simulink model "sim_5_dc_refer"  (R2022b)
settings: Solver=VariableStepAuto  StartTime=0.0  StopTime=10.0  RelTol=1e-3
model workspace: external: MAT-File dc_params.mat (data not in the file)
values from neighbouring files (symbols this model uses):
  b = 0.2    [dc_params.mat]    (also in sim_5_dc_param.m)
  J = 0.02    [dc_params.mat]    (also in sim_5_dc_param.m)
  K_e = 0.1    [dc_params.mat]    (also in sim_5_dc_param.m)
  K_t = 0.1    [dc_params.mat]    (also in sim_5_dc_param.m)
  L = 0.5    [dc_params.mat]    (also in sim_5_dc_param.m)
  R = 2    [dc_params.mat]    (also in sim_5_dc_param.m)
settings Model: ParameterArgumentNames=J,K_e,K_t,L,R,b  Creator=user  LastModifiedBy=user

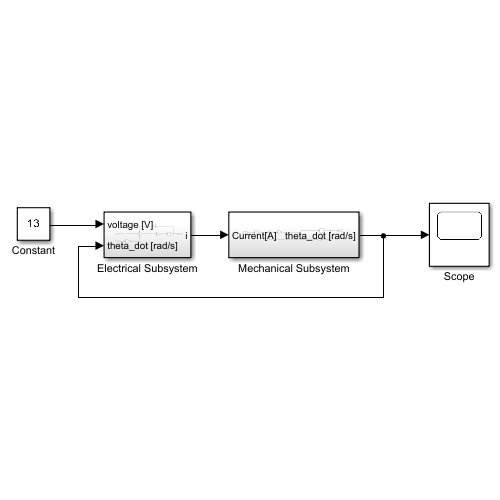
[thumbnail: Simulink's stored preview of the top-level diagram]
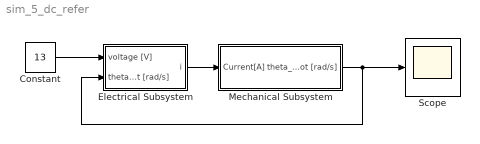
== system sim_5_dc_refer ==
  Constant : Constant  Value=13
  Electrical Subsystem : Subsystem
  Mechanical Subsystem : Subsystem
  Scope : Scope
  wires:
  Electrical Subsystem/1(i) -> Mechanical Subsystem/1(Current[A])
  Mechanical Subsystem/1(theta_dot [rad/s]) -> Electrical Subsystem/2(theta_dot [rad/s]), Scope/1
  Constant/1 -> Electrical Subsystem/1(voltage [V])

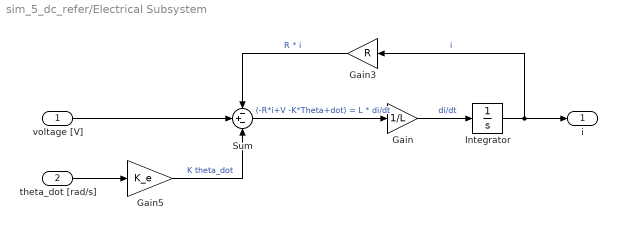
== system sim_5_dc_refer/Electrical Subsystem ==
  voltage [V] : Inport
  theta_dot [rad/s] : Inport  Port=2
  Gain : Gain  Gain=1/L
  Gain3 : Gain  Gain=R
  Gain5 : Gain  Gain=K_e
  Integrator : Integrator
  Sum : Sum  Inputs=-+-
  i : Outport
  wires:
  Gain/1 -> Integrator/1  "di/dt"
  Sum/1 -> Gain/1  "(-R*i+V -K*Theta+dot) = L * di/dt"
  Integrator/1 -> i/1, Gain3/1  "i"
  Gain3/1 -> Sum/1  "R * i"
  theta_dot [rad/s]/1 -> Gain5/1
  Gain5/1 -> Sum/3  "K theta_dot"
  voltage [V]/1 -> Sum/2

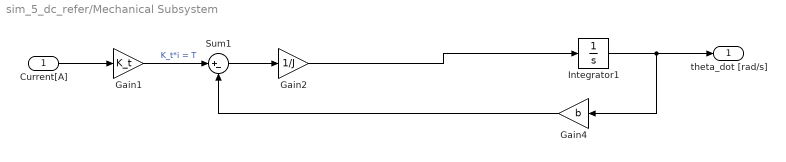
== system sim_5_dc_refer/Mechanical Subsystem ==
  Current[A] : Inport
  Gain1 : Gain  Gain=K_t
  Gain2 : Gain  Gain=1/J
  Gain4 : Gain  Gain=b
  Integrator1 : Integrator
  Sum1 : Sum  Inputs=|+-
  theta_dot [rad/s] : Outport
  wires:
  Integrator1/1 -> Gain4/1, theta_dot [rad/s]/1
  Gain2/1 -> Integrator1/1
  Gain4/1 -> Sum1/2
  Gain1/1 -> Sum1/1  "K_t*i = T"
  Sum1/1 -> Gain2/1
  Current[A]/1 -> Gain1/1
